simulink model "lineprotsys"  (Simulink 9.3)
settings: Solver=ode23tb  StartTime=0.0  StopTime=0.15  RelTol=1e-3  AbsTol=20e-6
values from neighbouring files (symbols this model uses):
  n = abs(fix(dif/360))    [DE_12.m]
undefined symbols (not defined in the file or in its folder): b, flagc, m, minx
libraries: elements x42, Relay_Elements x9
settings Model: Creator=Dr. Lotfifard  LastModifiedBy=renji  ExtModeTrigMode=oneshot  ExtModeArmWhenConnect=off
settings SolverCC: AutoScaleAbsTol=off  MaxOrder=2
settings DataIOCC: LimitDataPoints=on
settings OptimizationCC: BlockReduction=off  BooleanDataType=off  ExpressionDepthLimit=2147483647
settings DebuggingCC: SaveWithParameterizedLinksMsg=none  SignalResolutionControl=TryResolveAllWithWarning  MultiTaskDSMMsg=warning  MultiTaskCondExecSysMsg=none  StateNameClashWarn=warning
settings HardwareCC: TargetUnknown=on
settings RTWCC: TemplateMakefile=grt_unix.tmf
settings GRTTargetCC: GeneratePreprocessorConditionals=Disable all
settings SimscapeCC: SimscapeNormalizeSystem=off
settings ConfigurationSet: Description=SimMechanics 2G

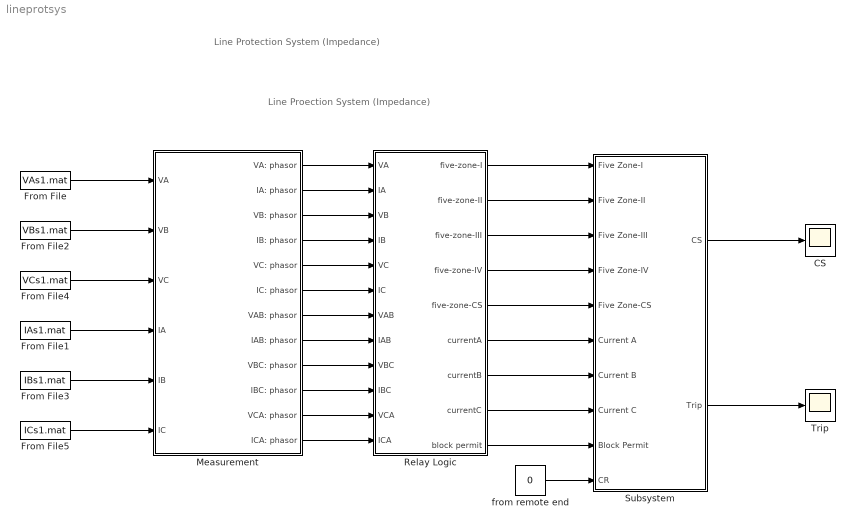
== system lineprotsys ==
  note: Line Protection System (Impedance)
  note: Line Proection System (Impedance)
  CS : Scope
  From File : FromFile  FileName=VAs1.mat  SampleTime=0
  From File1 : FromFile  FileName=IAs1.mat  SampleTime=0
  From File2 : FromFile  FileName=VBs1.mat  SampleTime=0
  From File3 : FromFile  FileName=IBs1.mat  SampleTime=0
  From File4 : FromFile  FileName=VCs1.mat  SampleTime=0
  From File5 : FromFile  FileName=ICs1.mat  SampleTime=0
  Measurement : Subsystem
  Relay Logic : Subsystem  mask{RelayZones=[70 90 100 120 60], fDetectZone=10, PolarZangle=pi/4, PolarZset=2, PowerSwingDetect=[0.05 1 2 5 10], ICtime=0.1, ICpu=0.005, CDang1=170, CDang2=0}
      mask prompts: RelayZones "Relay Zones [z1 z2 z3 z4 zb]"; fDetectZone "Fault Detection Zone (lenght and width)"; PolarZangle "Memory Polariztion: Zangle"; PolarZset "Memory Polariztion: Zsetting"; PowerSwingDetect "Power Swing Detection: [DeltT zs11 zs12 zs21 zs22"; ICtime "Inverse Current: time parameter"; ICpu "Inverse Current: pick up value"; CDang1 "Current Direction: angle1"; CDang2 "Current Direction: angle2"
  Subsystem : Subsystem
  Trip : Scope
  from remote end : Constant  Value=0
  wires:
  From File5/1 -> Measurement/6(IC)
  From File3/1 -> Measurement/5(IB)
  From File1/1 -> Measurement/4(IA)
  From File4/1 -> Measurement/3(VC)
  From File2/1 -> Measurement/2(VB)
  From File/1 -> Measurement/1(VA)
  Measurement/1(VA: phasor) -> Relay Logic/1(VA)
  Measurement/2(IA: phasor) -> Relay Logic/2(IA)
  Measurement/3(VB: phasor) -> Relay Logic/3(VB)
  Measurement/4(IB: phasor) -> Relay Logic/4(IB)
  Measurement/5(VC: phasor) -> Relay Logic/5(VC)
  Measurement/6(IC: phasor) -> Relay Logic/6(IC)
  Measurement/7(VAB: phasor) -> Relay Logic/7(VAB)
  Measurement/8(IAB: phasor) -> Relay Logic/8(IAB)
  Measurement/9(VBC: phasor) -> Relay Logic/9(VBC)
  Measurement/10(IBC: phasor) -> Relay Logic/10(IBC)
  Measurement/11(VCA: phasor) -> Relay Logic/11(VCA)
  Measurement/12(ICA: phasor) -> Relay Logic/12(ICA)
  Relay Logic/1(five-zone-I) -> Subsystem/1(Five Zone-I)
  Relay Logic/2(five-zone-II) -> Subsystem/2(Five Zone-II)
  Relay Logic/3(five-zone-III) -> Subsystem/3(Five Zone-III)
  Relay Logic/4(five-zone-IV) -> Subsystem/4(Five Zone-IV)
  Relay Logic/5(five-zone-CS) -> Subsystem/5(Five Zone-CS)
  Relay Logic/6(currentA) -> Subsystem/6(Current A)
  Relay Logic/7(currentB) -> Subsystem/7(Current B)
  Relay Logic/8(currentC) -> Subsystem/8(Current C)
  Relay Logic/9(block permit) -> Subsystem/9(Block Permit)
  from remote end/1 -> Subsystem/10(CR)
  Subsystem/1(CS) -> CS/1
  Subsystem/2(Trip) -> Trip/1

== system lineprotsys/Measurement ==
  note: Measurement Block
  VA : Inport
  VB : Inport  Port=2
  VC : Inport  Port=3
  IA : Inport  Port=4
  IB : Inport  Port=5
  IC : Inport  Port=6
  Input Signal Board : Subsystem
  Phase-phase Measurements : Subsystem
  Single Phase Measurements : Subsystem
  VA: phasor : Outport
  IA: phasor : Outport  Port=2
  VB: phasor : Outport  Port=3
  IB: phasor : Outport  Port=4
  VC: phasor : Outport  Port=5
  IC: phasor : Outport  Port=6
  VAB: phasor : Outport  Port=7
  IAB: phasor : Outport  Port=8
  VBC: phasor : Outport  Port=9
  IBC: phasor : Outport  Port=10
  VCA: phasor : Outport  Port=11
  ICA: phasor : Outport  Port=12
  wires:
  Phase-phase Measurements/1(VAB: phasor) -> VAB: phasor/1
  Phase-phase Measurements/6(ICA: phasor) -> ICA: phasor/1
  Phase-phase Measurements/4(IBC: phasor) -> IBC: phasor/1
  Phase-phase Measurements/2(IAB: phasor) -> IAB: phasor/1
  Phase-phase Measurements/3(VBC: phasor) -> VBC: phasor/1
  Phase-phase Measurements/5(VCA: phasor) -> VCA: phasor/1
  Single Phase Measurements/5(VC: phasor) -> VC: phasor/1
  Single Phase Measurements/6(IC: phasor) -> IC: phasor/1
  IC/1 -> Input Signal Board/6(IC)
  IB/1 -> Input Signal Board/5(IB)
  VC/1 -> Input Signal Board/3(VC)
  IA/1 -> Input Signal Board/4(IA)
  Single Phase Measurements/2(IA: phasor) -> IA: phasor/1
  Single Phase Measurements/3(VB: phasor) -> VB: phasor/1
  Single Phase Measurements/4(IB: phasor) -> IB: phasor/1
  VA/1 -> Input Signal Board/1(VA)
  Single Phase Measurements/1(VA: phasor) -> VA: phasor/1
  VB/1 -> Input Signal Board/2(VB)

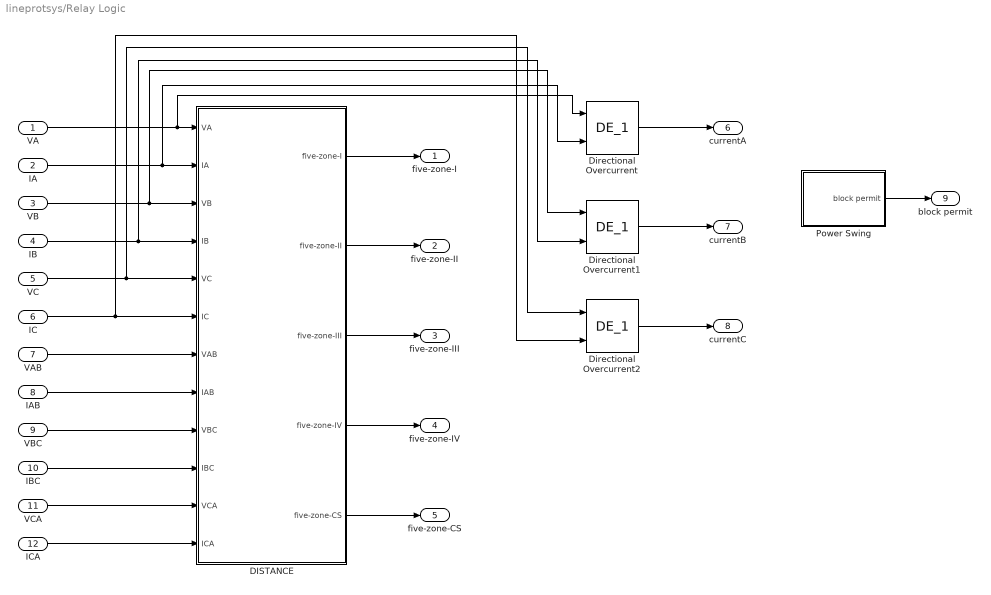
== system lineprotsys/Relay Logic ==
  VA : Inport
  IA : Inport  Port=2
  VB : Inport  Port=3
  IB : Inport  Port=4
  VC : Inport  Port=5
  IC : Inport  Port=6
  VAB : Inport  Port=7
  IAB : Inport  Port=8
  VBC : Inport  Port=9
  IBC : Inport  Port=10
  VCA : Inport  Port=11
  ICA : Inport  Port=12
  "  Directional Overcurrent" : Relay_Elements/  DE_1  alpha=CDang1  beta=CDang2  fs=20*60
  "  Directional Overcurrent1" : Relay_Elements/  DE_1  alpha=CDang1  beta=CDang2  fs=20*60
  "  Directional Overcurrent2" : Relay_Elements/  DE_1  alpha=CDang1  beta=CDang2  fs=20*60
  DISTANCE : Subsystem
  Power Swing : Subsystem  mask{Tswing=PowerSwingDetect(1)}
      mask prompts: Tswing "T Power Swing (sec)"
  five-zone-I : Outport
  five-zone-II : Outport  Port=2
  five-zone-III : Outport  Port=3
  five-zone-IV : Outport  Port=4
  five-zone-CS : Outport  Port=5
  currentA : Outport  Port=6
  currentB : Outport  Port=7
  currentC : Outport  Port=8
  block permit : Outport  Port=9
  wires:
  DISTANCE/1(five-zone-I) -> five-zone-I/1
  DISTANCE/2(five-zone-II) -> five-zone-II/1
  DISTANCE/3(five-zone-III) -> five-zone-III/1
  DISTANCE/4(five-zone-IV) -> five-zone-IV/1
  DISTANCE/5(five-zone-CS) -> five-zone-CS/1
  "  Directional Overcurrent1"/1 -> currentB/1
  "  Directional Overcurrent"/1 -> currentA/1
  "  Directional Overcurrent2"/1 -> currentC/1
  Power Swing/1(block permit) -> block permit/1
  VA/1 -> "  Directional Overcurrent"/1, DISTANCE/1(VA)
  VB/1 -> "  Directional Overcurrent1"/1, DISTANCE/3(VB)
  IB/1 -> "  Directional Overcurrent1"/2, DISTANCE/4(IB)
  VC/1 -> "  Directional Overcurrent2"/1, DISTANCE/5(VC)
  IC/1 -> "  Directional Overcurrent2"/2, DISTANCE/6(IC)
  VAB/1 -> DISTANCE/7(VAB)
  IAB/1 -> DISTANCE/8(IAB)
  VBC/1 -> DISTANCE/9(VBC)
  IBC/1 -> DISTANCE/10(IBC)
  VCA/1 -> DISTANCE/11(VCA)
  ICA/1 -> DISTANCE/12(ICA)
  IA/1 -> "  Directional Overcurrent"/2, DISTANCE/2(IA)

== system lineprotsys/Subsystem ==
  Five Zone-I : Inport
  Five Zone-II : Inport  Port=2
  Five Zone-III : Inport  Port=3
  Five Zone-IV : Inport  Port=4
  Five Zone-CS : Inport  Port=5
  Current A : Inport  Port=6
  Current B : Inport  Port=7
  Current C : Inport  Port=8
  Block Permit : Inport  Port=9
  CR : Inport  Port=10
  1 : Logic  Operator=OR  Inputs=4  AllPortsSameDT=off
  2 : Logic  Inputs=4
  3 : Logic  Operator=OR  Inputs=3  AllPortsSameDT=off
  4 : Logic  Operator=OR
  Not : Logic  Operator=NOT  AllPortsSameDT=off  OutDataTypeStr=boolean
  Not1 : Logic  Operator=NOT  AllPortsSameDT=off  OutDataTypeStr=boolean
  Not2 : Logic  Operator=NOT  AllPortsSameDT=off  OutDataTypeStr=boolean
  CS : Outport
  Trip : Outport  Port=2
  wires:
  Five Zone-II/1 -> 1/2
  Five Zone-IV/1 -> 1/4
  Five Zone-I/1 -> 1/1
  Current A/1 -> 3/1
  Current C/1 -> 3/3
  3/1 -> 4/2
  Five Zone-III/1 -> 1/3
  Current B/1 -> 3/2
  1/1 -> 4/1
  Block Permit/1 -> Not/1
  CR/1 -> Not2/1
  Not2/1 -> 2/4
  Not/1 -> 2/3
  Five Zone-CS/1 -> Not1/1
  Not1/1 -> CS/1, 2/2
  2/1 -> Trip/1
  4/1 -> 2/1

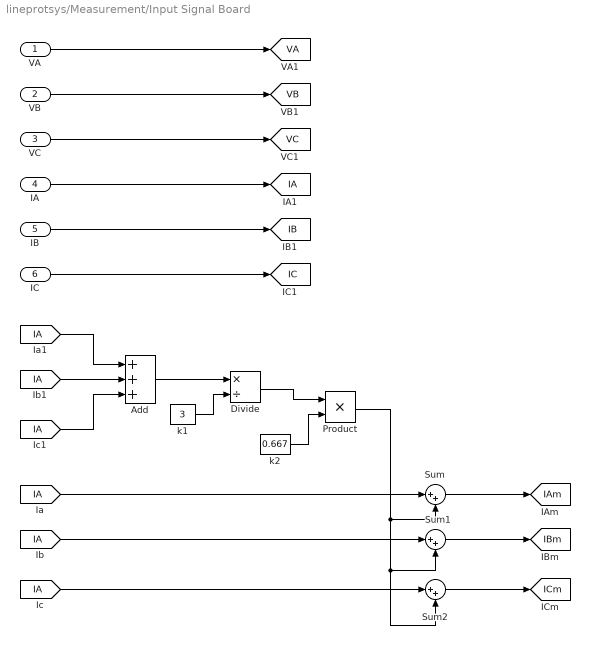
== system lineprotsys/Measurement/Input Signal Board ==
  VA : Inport
  VB : Inport  Port=2
  VC : Inport  Port=3
  IA : Inport  Port=4
  IB : Inport  Port=5
  IC : Inport  Port=6
  Add : Sum  Inputs=+++
  Divide : Product  Inputs=*/
  Product : Product
  Sum : Sum  Inputs=|++
  Sum1 : Sum  Inputs=|++
  Sum2 : Sum  Inputs=|++
  k1 : Constant  Value=3
  k2 : Constant  Value=0.667
  tag scope: IA=global, IAm=global, IB=global, IBm=global, IC=global, ICm=global, VA=global, VB=global, VC=global
  wires:
  Add/1 -> Divide/1
  k1/1 -> Divide/2
  Divide/1 -> Product/1
  VC/1 -> [VC]
  k2/1 -> Product/2
  VB/1 -> [VB]
  IA/1 -> [IA]
  IB/1 -> [IB]
  IC/1 -> [IC]
  [IA] -> Add/2
  [IA] -> Add/1
  [IA] -> Add/3
  VA/1 -> [VA]
  Sum2/1 -> [ICm]
  Sum1/1 -> [IBm]
  Sum/1 -> [IAm]
  [IA] -> Sum2/1
  [IA] -> Sum1/1
  [IA] -> Sum/1
  Product/1 -> Sum/2, Sum1/2, Sum2/2

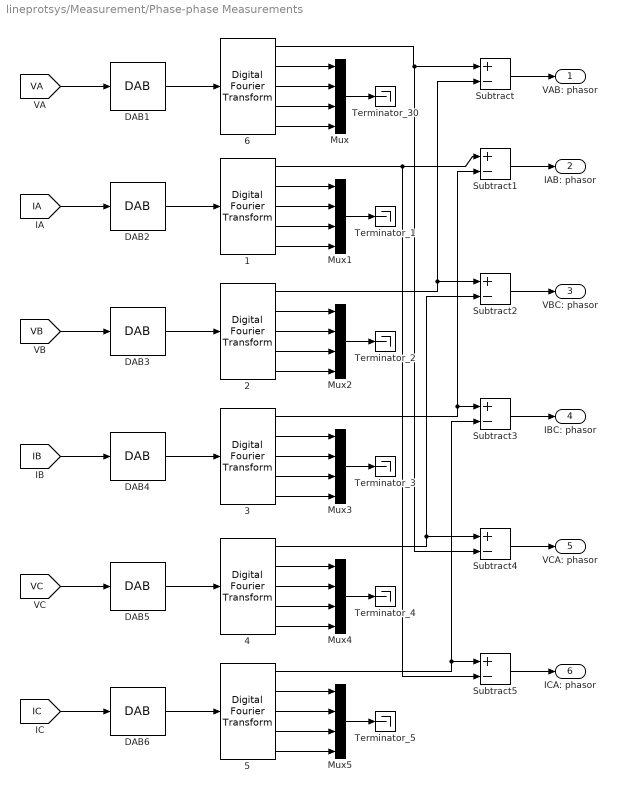
== system lineprotsys/Measurement/Phase-phase Measurements ==
   {1..6} (6 alike) : elements/   fo=60  window_size=32  harmonic=[1 2 3 4 5]
  DAB{1..6} (6 alike) : elements/DAB  filter=off  approx=Bessel  order=2  numerator=[]  denominator=[]  freq=360  resdis=off  vertres=12  xmax=10  winsize=32  G=1.0  fs=60*32
  Mux{,1..5} (6 alike) : Mux
  Subtract{,1..5} (6 alike) : Sum  Inputs=+-
  Terminator_{1..5,30} (6 alike) : Terminator
  VAB: phasor : Outport
  IAB: phasor : Outport  Port=2
  VBC: phasor : Outport  Port=3
  IBC: phasor : Outport  Port=4
  VCA: phasor : Outport  Port=5
  ICA: phasor : Outport  Port=6
  wires:
  " 4"/5 -> Mux4/4
  Mux4/1 -> Terminator_4/1
  DAB5/1 -> " 4"/1
  " 2"/3 -> Mux2/2
  " 2"/2 -> Mux2/1
  " 2"/5 -> Mux2/4
  DAB3/1 -> " 2"/1
  " 2"/4 -> Mux2/3
  Mux2/1 -> Terminator_2/1
  " 4"/2 -> Mux4/1
  " 4"/3 -> Mux4/2
  " 4"/4 -> Mux4/3
  " 1"/2 -> Mux1/1
  " 1"/3 -> Mux1/2
  " 1"/4 -> Mux1/3
  " 1"/5 -> Mux1/4
  Mux1/1 -> Terminator_1/1
  DAB2/1 -> " 1"/1
  DAB1/1 -> " 6"/1
  " 5"/3 -> Mux5/2
  " 5"/2 -> Mux5/1
  " 5"/4 -> Mux5/3
  " 5"/5 -> Mux5/4
  Mux5/1 -> Terminator_5/1
  DAB6/1 -> " 5"/1
  " 6"/5 -> Mux/4
  " 6"/3 -> Mux/2
  Mux/1 -> Terminator_30/1
  Mux3/1 -> Terminator_3/1
  " 3"/3 -> Mux3/2
  DAB4/1 -> " 3"/1
  " 3"/2 -> Mux3/1
  " 3"/4 -> Mux3/3
  " 3"/5 -> Mux3/4
  " 6"/4 -> Mux/3
  " 6"/2 -> Mux/1
  [VA] -> DAB1/1
  [IA] -> DAB2/1
  [VB] -> DAB3/1
  [IB] -> DAB4/1
  [VC] -> DAB5/1
  [IC] -> DAB6/1
  " 6"/1 -> Subtract4/2, Subtract/1
  " 2"/1 -> Subtract2/1, Subtract/2
  Subtract/1 -> VAB: phasor/1
  " 1"/1 -> Subtract5/2, Subtract1/1
  " 3"/1 -> Subtract3/1, Subtract1/2
  " 4"/1 -> Subtract4/1, Subtract2/2
  Subtract2/1 -> VBC: phasor/1
  Subtract1/1 -> IAB: phasor/1
  Subtract3/1 -> IBC: phasor/1
  Subtract4/1 -> VCA: phasor/1
  Subtract5/1 -> ICA: phasor/1
  " 5"/1 -> Subtract5/1, Subtract3/2

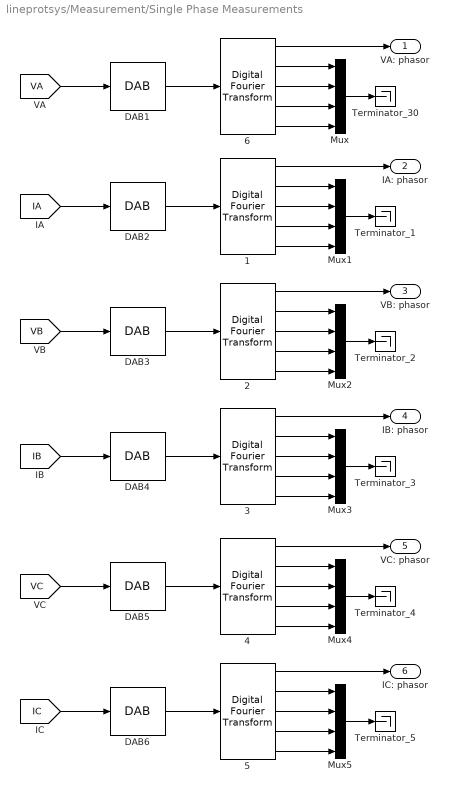
== system lineprotsys/Measurement/Single Phase Measurements ==
   {1..6} (6 alike) : elements/   fo=60  window_size=32  harmonic=[1 2 3 4 5]
  DAB{1..6} (6 alike) : elements/DAB  filter=off  approx=Bessel  order=2  numerator=[]  denominator=[]  freq=360  resdis=off  vertres=12  xmax=10  winsize=32  G=1.0  fs=60*32
  Mux{,1..5} (6 alike) : Mux
  Terminator_{1..5,30} (6 alike) : Terminator
  VA: phasor : Outport
  IA: phasor : Outport  Port=2
  VB: phasor : Outport  Port=3
  IB: phasor : Outport  Port=4
  VC: phasor : Outport  Port=5
  IC: phasor : Outport  Port=6
  wires:
  " 4"/1 -> VC: phasor/1
  " 4"/5 -> Mux4/4
  Mux4/1 -> Terminator_4/1
  DAB5/1 -> " 4"/1
  " 2"/3 -> Mux2/2
  " 2"/2 -> Mux2/1
  " 2"/5 -> Mux2/4
  DAB3/1 -> " 2"/1
  " 2"/4 -> Mux2/3
  " 2"/1 -> VB: phasor/1
  Mux2/1 -> Terminator_2/1
  " 4"/2 -> Mux4/1
  " 4"/3 -> Mux4/2
  " 4"/4 -> Mux4/3
  " 1"/2 -> Mux1/1
  " 1"/3 -> Mux1/2
  " 1"/4 -> Mux1/3
  " 1"/5 -> Mux1/4
  Mux1/1 -> Terminator_1/1
  " 1"/1 -> IA: phasor/1
  DAB2/1 -> " 1"/1
  DAB1/1 -> " 6"/1
  " 5"/1 -> IC: phasor/1
  " 5"/3 -> Mux5/2
  " 5"/2 -> Mux5/1
  " 5"/4 -> Mux5/3
  " 5"/5 -> Mux5/4
  Mux5/1 -> Terminator_5/1
  DAB6/1 -> " 5"/1
  " 6"/5 -> Mux/4
  " 6"/3 -> Mux/2
  Mux/1 -> Terminator_30/1
  Mux3/1 -> Terminator_3/1
  " 3"/3 -> Mux3/2
  " 3"/1 -> IB: phasor/1
  DAB4/1 -> " 3"/1
  " 6"/1 -> VA: phasor/1
  " 3"/2 -> Mux3/1
  " 3"/4 -> Mux3/3
  " 3"/5 -> Mux3/4
  " 6"/4 -> Mux/3
  " 6"/2 -> Mux/1
  [VA] -> DAB1/1
  [IA] -> DAB2/1
  [VB] -> DAB3/1
  [IB] -> DAB4/1
  [VC] -> DAB5/1
  [IC] -> DAB6/1

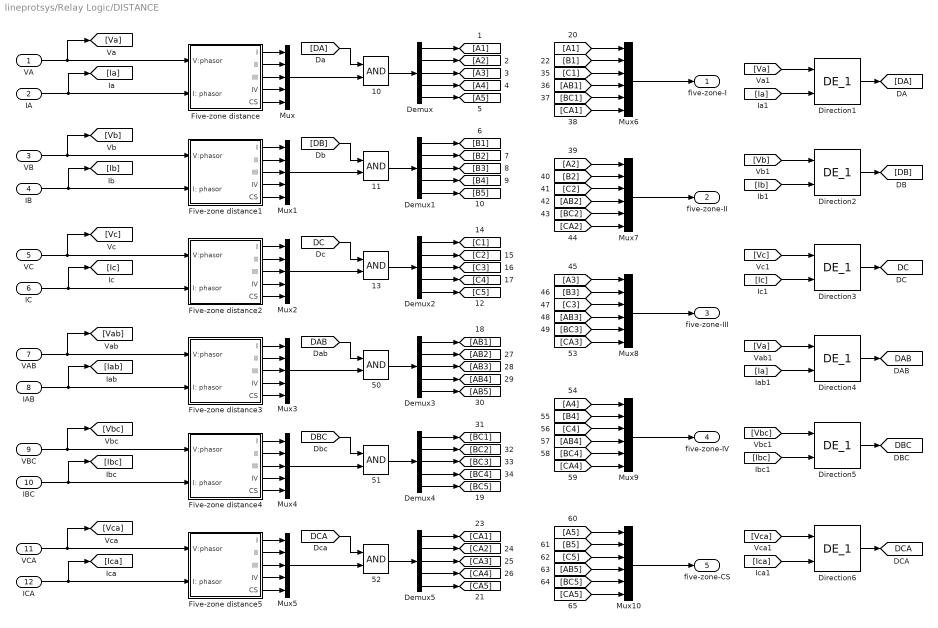
== system lineprotsys/Relay Logic/DISTANCE ==
  VA : Inport
  IA : Inport  Port=2
  VB : Inport  Port=3
  IB : Inport  Port=4
  VC : Inport  Port=5
  IC : Inport  Port=6
  VAB : Inport  Port=7
  IAB : Inport  Port=8
  VBC : Inport  Port=9
  IBC : Inport  Port=10
  VCA : Inport  Port=11
  ICA : Inport  Port=12
    Direction{1..6} (6 alike) : Relay_Elements/  DE_1  alpha=CDang1  beta=CDang2  fs=20*60
  "10 " : Logic
  {11,13,50..52} (5 alike) : Logic
  Demux{,1..5} (6 alike) : Demux  Outputs=5
  Five-zone distance : Subsystem
  Five-zone distance1 : Subsystem
  Five-zone distance2 : Subsystem
  Five-zone distance3 : Subsystem
  Five-zone distance4 : Subsystem
  Five-zone distance5 : Subsystem
  Mux{,1..5} (6 alike) : Mux  Inputs=5
  Mux{6..10} (5 alike) : Mux  Inputs=6
  five-zone-I : Outport
  five-zone-II : Outport  Port=2
  five-zone-III : Outport  Port=3
  five-zone-IV : Outport  Port=4
  five-zone-CS : Outport  Port=5
  tag scope: DAB=global, DBC=global, DC=global, DCA=global
  wires:
  VB/1 -> Five-zone distance1/1(V:phasor), [Vb]
  IB/1 -> Five-zone distance1/2(I: phasor), [Ib]
  [DB] -> 11/1
  Demux1/1 -> [B1]
  Demux1/3 -> [B3]
  Five-zone distance1/4(IV) -> Mux1/4
  Five-zone distance1/5(CS) -> Mux1/5
  Mux1/1 -> 11/2
  Demux1/2 -> [B2]
  Demux1/5 -> [B5]
  Five-zone distance1/1(I) -> Mux1/1
  Five-zone distance1/3(III) -> Mux1/3
  11/1 -> Demux1/1
  Five-zone distance1/2(II) -> Mux1/2
  Demux1/4 -> [B4]
  Five-zone distance/2(II) -> Mux/2
  Five-zone distance/5(CS) -> Mux/5
  Five-zone distance/4(IV) -> Mux/4
  "  Direction1"/1 -> [DA]
  Five-zone distance/1(I) -> Mux/1
  IA/1 -> [Ia], Five-zone distance/2(I: phasor)
  VA/1 -> [Va], Five-zone distance/1(V:phasor)
  Demux/3 -> [A3]
  Demux/5 -> [A5]
  Demux/4 -> [A4]
  [B2] -> Mux7/2
  [AB2] -> Mux7/4
  [C2] -> Mux7/3
  [CA2] -> Mux7/6
  [A2] -> Mux7/1
  Mux7/1 -> five-zone-II/1
  [BC2] -> Mux7/5
  [B1] -> Mux6/2
  [CA1] -> Mux6/6
  "10 "/1 -> Demux/1
  [BC1] -> Mux6/5
  [A1] -> Mux6/1
  Demux/1 -> [A1]
  Demux/2 -> [A2]
  [C1] -> Mux6/3
  [AB1] -> Mux6/4
  [A3] -> Mux8/1
  [B3] -> Mux8/2
  [C3] -> Mux8/3
  [CA3] -> Mux8/6
  [AB3] -> Mux8/4
  [BC3] -> Mux8/5
  Mux8/1 -> five-zone-III/1
  Mux10/1 -> five-zone-CS/1
  [A5] -> Mux10/1
  [C5] -> Mux10/3
  [CA5] -> Mux10/6
  [B5] -> Mux10/2
  [BC5] -> Mux10/5
  [AB5] -> Mux10/4
  [B4] -> Mux9/2
  [CA4] -> Mux9/6
  [BC4] -> Mux9/5
  [AB4] -> Mux9/4
  [A4] -> Mux9/1
  [C4] -> Mux9/3
  Mux9/1 -> five-zone-IV/1
  Mux2/1 -> 13/2
  Demux2/3 -> [C3]
  Five-zone distance2/1(I) -> Mux2/1
  Demux2/1 -> [C1]
  VC/1 -> Five-zone distance2/1(V:phasor), [Vc]
  Five-zone distance2/3(III) -> Mux2/3
  IC/1 -> Five-zone distance2/2(I: phasor), [Ic]
  [DC] -> 13/1
  Five-zone distance2/5(CS) -> Mux2/5
  Five-zone distance2/2(II) -> Mux2/2
  13/1 -> Demux2/1
  Five-zone distance2/4(IV) -> Mux2/4
  Demux2/2 -> [C2]
  Demux2/5 -> [C5]
  Demux2/4 -> [C4]
  Five-zone distance/3(III) -> Mux/3
  [DA] -> "10 "/1
  Mux/1 -> "10 "/2
  Five-zone distance5/4(IV) -> Mux5/4
  Mux5/1 -> 52/2
  IAB/1 -> Five-zone distance3/2(I: phasor), [Iab]
  Five-zone distance3/1(I) -> Mux3/1
  Demux4/5 -> [BC5]
  Demux4/4 -> [BC4]
  Demux3/5 -> [AB5]
  Five-zone distance3/3(III) -> Mux3/3
  Demux3/4 -> [AB4]
  Five-zone distance5/5(CS) -> Mux5/5
  [DCA] -> 52/1
  Demux5/5 -> [CA5]
  Demux3/1 -> [AB1]
  Five-zone distance3/4(IV) -> Mux3/4
  Five-zone distance3/5(CS) -> Mux3/5
  [DAB] -> 50/1
  Demux3/3 -> [AB3]
  IBC/1 -> Five-zone distance4/2(I: phasor), [Ibc]
  Mux4/1 -> 51/2
  50/1 -> Demux3/1
  Demux4/1 -> [BC1]
  Five-zone distance5/1(I) -> Mux5/1
  52/1 -> Demux5/1
  Demux5/1 -> [CA1]
  51/1 -> Demux4/1
  VAB/1 -> Five-zone distance3/1(V:phasor), [Vab]
  Demux4/3 -> [BC3]
  Demux4/2 -> [BC2]
  Five-zone distance3/2(II) -> Mux3/2
  VBC/1 -> Five-zone distance4/1(V:phasor), [Vbc]
  Mux3/1 -> 50/2
  Demux3/2 -> [AB2]
  Five-zone distance5/2(II) -> Mux5/2
  ICA/1 -> Five-zone distance5/2(I: phasor), [Ica]
  Demux5/2 -> [CA2]
  Five-zone distance5/3(III) -> Mux5/3
  Demux5/3 -> [CA3]
  [DBC] -> 51/1
  Demux5/4 -> [CA4]
  VCA/1 -> Five-zone distance5/1(V:phasor), [Vca]
  [Va] -> "  Direction4"/1
  "  Direction4"/1 -> [DAB]
  [Ia] -> "  Direction4"/2
  [Ica] -> "  Direction6"/2
  [Vca] -> "  Direction6"/1
  "  Direction6"/1 -> [DCA]
  [Va] -> "  Direction1"/1
  [Ia] -> "  Direction1"/2
  [Vc] -> "  Direction3"/1
  [Ic] -> "  Direction3"/2
  "  Direction3"/1 -> [DC]
  [Vbc] -> "  Direction5"/1
  "  Direction5"/1 -> [DBC]
  [Ibc] -> "  Direction5"/2
  Mux6/1 -> five-zone-I/1
  "  Direction2"/1 -> [DB]
  [Ib] -> "  Direction2"/2
  [Vb] -> "  Direction2"/1
  Five-zone distance4/1(I) -> Mux4/1
  Five-zone distance4/2(II) -> Mux4/2
  Five-zone distance4/3(III) -> Mux4/3
  Five-zone distance4/4(IV) -> Mux4/4
  Five-zone distance4/5(CS) -> Mux4/5

== system lineprotsys/Relay Logic/Power Swing ==
  " 3" : Terminator
  " 4" : Terminator
  " 6" : Terminator
  4 : Logic  Operator=OR
  Subsystem : Subsystem
  Z: power swing : Subsystem  mask(Zone Comparator){typez=Free expression, z1=[0.2 0.2;-0.2 0.2; -0.2 -0.2;0.2 -0.2], z2=[0 0;1 1; -1 1;0 0], z3=[1 1;-1 1;-1 -1;1 -1], z4=[0 0;0 0;0 0;0 0], zr=[0 0;0 0;0 0;0 0], fs=32*60}
      mask prompts: typez "shape"; z1 "Zone 1"; z2 "Zone 2"; z3 "Zone 3"; z4 "Zone 4"; zr "Reverse Zone"; fs "Sampling frecuency (Hz):"
      mask help: This block performs the zone comparison. Its inputs are the resistance and reactance signals. Four forward and one backward zones are implemented. The output that corresponds to the zone where the impedance is located is set to one while the rest of the outputs are zero Either the mho or free expression characteristics may be set. For the mho characteristic, the zones are defined by specifying the center of each circle (all the circles are tangent to the origin). For the free expression, arrays with consecutive vertices specify the polygons for each zone.
      mask init:
      | zc1;
      mask Help: web(['file:///' which('zc.html')]);
      mask TypeOptions typez: Mho characteristic | Free expression
      mask Display:
      | plot(x1(:,1),x1(:,2));
      | plot(x2(:,1),x2(:,2));
      | plot(x3(:,1),x3(:,2));
      | plot(x4(:,1),x4(:,2));
      | plot(xr(:,1),xr(:,2));
  block permit : Outport
  wires:
  Z: power swing/3(3) -> " 3"/1
  Z: power swing/2(2) -> 4/2
  Z: power swing/1(1) -> Subsystem/1(Z1), 4/1
  [ZA] -> Z: power swing/1(Z)
  Z: power swing/5(R) -> " 6"/1
  Z: power swing/4(4) -> " 4"/1
  4/1 -> Subsystem/2(Z2)
  Subsystem/1(block) -> block permit/1

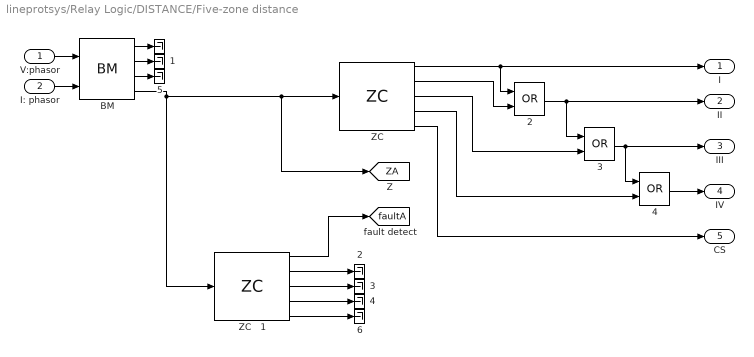
== system lineprotsys/Relay Logic/DISTANCE/Five-zone distance ==
  V:phasor : Inport
  I: phasor : Inport  Port=2
   {,1..6} (7 alike) : Terminator
  "2 " : Logic  Operator=OR
  3 : Logic  Operator=OR
  4 : Logic  Operator=OR
  BM : elements/BM  tpostv=none  plenv=4  tposti=none  pleni=4  tposts=none  plens=4  tpostz=none  plenz=4
  "ZC   " : elements/ZC     typez=Free expression  z1="[0  0; RelayZones(1) 0; RelayZones(1) RelayZones(1); 0 RelayZones(1)]"  z2="[0  0; RelayZones(2) 0; RelayZones(2) RelayZones(2); 0 RelayZones(2)]"  z3="[0  0; RelayZones(3) 0; RelayZones(3) RelayZones(3); 0 RelayZones(3)]"  z4="[0  0; RelayZones(4) 0; RelayZones(4) RelayZones(4); 0 RelayZones(4)]"  zr="[0  0; -RelayZones(5) 0; -RelayZones(5) -RelayZones(5); 0 -RelayZones(5)]"  fs=32*60
  ZC   1 : elements/ZC     typez=Free expression  z1="[0  0; RelayZones(1) 0; RelayZones(1) RelayZones(1); 0 RelayZones(1)]"  z2="[0  0; RelayZones(2) 0; RelayZones(2) RelayZones(2); 0 RelayZones(2)]"  z3="[0  0; RelayZones(3) 0; RelayZones(3) RelayZones(3); 0 RelayZones(3)]"  z4="[0  0; RelayZones(4) 0; RelayZones(4) RelayZones(4); 0 RelayZones(4)]"  zr="[0  0; -RelayZones(5) 0; -RelayZones(5) -RelayZones(5); 0 -RelayZones(5)]"  fs=32*60
  I : Outport
  II : Outport  Port=2
  III : Outport  Port=3
  IV : Outport  Port=4
  CS : Outport  Port=5
  tag scope: ZA=global, faultA=global
  wires:
  BM/1 -> " "/1
  BM/2 -> " 1"/1
  BM/3 -> " 5"/1
  V:phasor/1 -> BM/1
  I: phasor/1 -> BM/2
  BM/4 -> ZC   1/1, [ZA], "ZC   "/1
  ZC   1/2 -> " 2"/1
  ZC   1/3 -> " 3"/1
  ZC   1/4 -> " 4"/1
  ZC   1/5 -> " 6"/1
  "2 "/1 -> II/1, 3/1
  3/1 -> 4/1, III/1
  4/1 -> IV/1
  "ZC   "/5 -> CS/1
  "ZC   "/4 -> 4/2
  "ZC   "/3 -> 3/2
  "ZC   "/2 -> "2 "/2
  "ZC   "/1 -> "2 "/1, I/1
  ZC   1/1 -> [faultA]

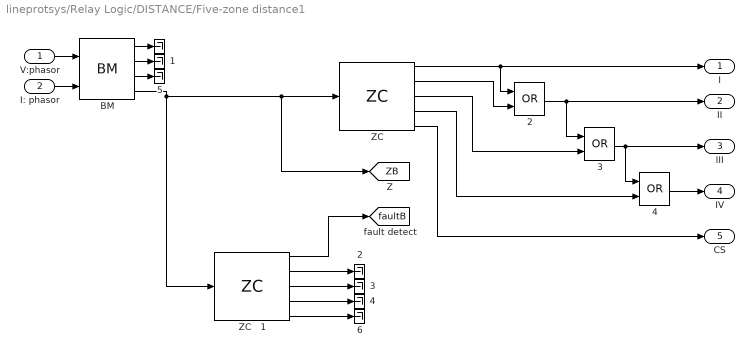
== system lineprotsys/Relay Logic/DISTANCE/Five-zone distance1 ==
  V:phasor : Inport
  I: phasor : Inport  Port=2
   {,1..6} (7 alike) : Terminator
  "2 " : Logic  Operator=OR
  3 : Logic  Operator=OR
  4 : Logic  Operator=OR
  BM : elements/BM  tpostv=none  plenv=4  tposti=none  pleni=4  tposts=none  plens=4  tpostz=none  plenz=4
  "ZC   " : elements/ZC     typez=Free expression  z1="[0  0; RelayZones(1) 0; RelayZones(1) RelayZones(1); 0 RelayZones(1)]"  z2="[0  0; RelayZones(2) 0; RelayZones(2) RelayZones(2); 0 RelayZones(2)]"  z3="[0  0; RelayZones(3) 0; RelayZones(3) RelayZones(3); 0 RelayZones(3)]"  z4="[0  0; RelayZones(4) 0; RelayZones(4) RelayZones(4); 0 RelayZones(4)]"  zr="[0  0; -RelayZones(5) 0; -RelayZones(5) -RelayZones(5); 0 -RelayZones(5)]"  fs=32*60
  ZC   1 : elements/ZC     typez=Free expression  z1="[0  0; RelayZones(1) 0; RelayZones(1) RelayZones(1); 0 RelayZones(1)]"  z2="[0  0; RelayZones(2) 0; RelayZones(2) RelayZones(2); 0 RelayZones(2)]"  z3="[0  0; RelayZones(3) 0; RelayZones(3) RelayZones(3); 0 RelayZones(3)]"  z4="[0  0; RelayZones(4) 0; RelayZones(4) RelayZones(4); 0 RelayZones(4)]"  zr="[0  0; -RelayZones(5) 0; -RelayZones(5) -RelayZones(5); 0 -RelayZones(5)]"  fs=32*60
  I : Outport
  II : Outport  Port=2
  III : Outport  Port=3
  IV : Outport  Port=4
  CS : Outport  Port=5
  tag scope: ZB=global, faultB=global
  wires:
  BM/1 -> " "/1
  BM/2 -> " 1"/1
  BM/3 -> " 5"/1
  V:phasor/1 -> BM/1
  I: phasor/1 -> BM/2
  BM/4 -> ZC   1/1, [ZB], "ZC   "/1
  ZC   1/2 -> " 2"/1
  ZC   1/3 -> " 3"/1
  ZC   1/4 -> " 4"/1
  ZC   1/5 -> " 6"/1
  "2 "/1 -> II/1, 3/1
  3/1 -> 4/1, III/1
  4/1 -> IV/1
  "ZC   "/5 -> CS/1
  "ZC   "/4 -> 4/2
  "ZC   "/3 -> 3/2
  "ZC   "/2 -> "2 "/2
  "ZC   "/1 -> "2 "/1, I/1
  ZC   1/1 -> [faultB]

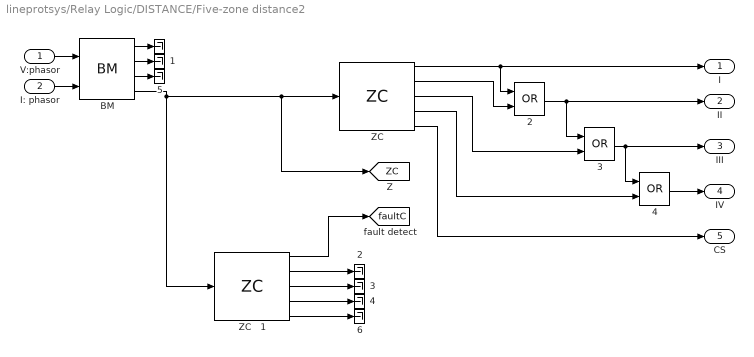
== system lineprotsys/Relay Logic/DISTANCE/Five-zone distance2 ==
  V:phasor : Inport
  I: phasor : Inport  Port=2
   {,1..6} (7 alike) : Terminator
  "2 " : Logic  Operator=OR
  3 : Logic  Operator=OR
  4 : Logic  Operator=OR
  BM : elements/BM  tpostv=none  plenv=4  tposti=none  pleni=4  tposts=none  plens=4  tpostz=none  plenz=4
  "ZC   " : elements/ZC     typez=Free expression  z1="[0  0; RelayZones(1) 0; RelayZones(1) RelayZones(1); 0 RelayZones(1)]"  z2="[0  0; RelayZones(2) 0; RelayZones(2) RelayZones(2); 0 RelayZones(2)]"  z3="[0  0; RelayZones(3) 0; RelayZones(3) RelayZones(3); 0 RelayZones(3)]"  z4="[0  0; RelayZones(4) 0; RelayZones(4) RelayZones(4); 0 RelayZones(4)]"  zr="[0  0; -RelayZones(5) 0; -RelayZones(5) -RelayZones(5); 0 -RelayZones(5)]"  fs=32*60
  ZC   1 : elements/ZC     typez=Free expression  z1="[0  0; RelayZones(1) 0; RelayZones(1) RelayZones(1); 0 RelayZones(1)]"  z2="[0  0; RelayZones(2) 0; RelayZones(2) RelayZones(2); 0 RelayZones(2)]"  z3="[0  0; RelayZones(3) 0; RelayZones(3) RelayZones(3); 0 RelayZones(3)]"  z4="[0  0; RelayZones(4) 0; RelayZones(4) RelayZones(4); 0 RelayZones(4)]"  zr="[0  0; -RelayZones(5) 0; -RelayZones(5) -RelayZones(5); 0 -RelayZones(5)]"  fs=32*60
  I : Outport
  II : Outport  Port=2
  III : Outport  Port=3
  IV : Outport  Port=4
  CS : Outport  Port=5
  tag scope: ZC=global, faultC=global
  wires:
  BM/1 -> " "/1
  BM/2 -> " 1"/1
  BM/3 -> " 5"/1
  V:phasor/1 -> BM/1
  I: phasor/1 -> BM/2
  BM/4 -> ZC   1/1, [ZC], "ZC   "/1
  ZC   1/2 -> " 2"/1
  ZC   1/3 -> " 3"/1
  ZC   1/4 -> " 4"/1
  ZC   1/5 -> " 6"/1
  "2 "/1 -> II/1, 3/1
  3/1 -> 4/1, III/1
  4/1 -> IV/1
  "ZC   "/5 -> CS/1
  "ZC   "/4 -> 4/2
  "ZC   "/3 -> 3/2
  "ZC   "/2 -> "2 "/2
  "ZC   "/1 -> "2 "/1, I/1
  ZC   1/1 -> [faultC]

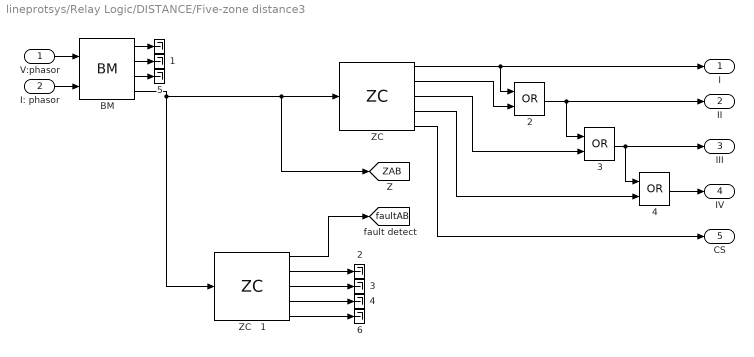
== system lineprotsys/Relay Logic/DISTANCE/Five-zone distance3 ==
  V:phasor : Inport
  I: phasor : Inport  Port=2
   {,1..6} (7 alike) : Terminator
  "2 " : Logic  Operator=OR
  3 : Logic  Operator=OR
  4 : Logic  Operator=OR
  BM : elements/BM  tpostv=none  plenv=4  tposti=none  pleni=4  tposts=none  plens=4  tpostz=none  plenz=4
  "ZC   " : elements/ZC     typez=Free expression  z1="[0  0; RelayZones(1) 0; RelayZones(1) RelayZones(1); 0 RelayZones(1)]"  z2="[0  0; RelayZones(2) 0; RelayZones(2) RelayZones(2); 0 RelayZones(2)]"  z3="[0  0; RelayZones(3) 0; RelayZones(3) RelayZones(3); 0 RelayZones(3)]"  z4="[0  0; RelayZones(4) 0; RelayZones(4) RelayZones(4); 0 RelayZones(4)]"  zr="[0  0; -RelayZones(5) 0; -RelayZones(5) -RelayZones(5); 0 -RelayZones(5)]"  fs=32*60
  ZC   1 : elements/ZC     typez=Free expression  z1="[0  0; RelayZones(1) 0; RelayZones(1) RelayZones(1); 0 RelayZones(1)]"  z2="[0  0; RelayZones(2) 0; RelayZones(2) RelayZones(2); 0 RelayZones(2)]"  z3="[0  0; RelayZones(3) 0; RelayZones(3) RelayZones(3); 0 RelayZones(3)]"  z4="[0  0; RelayZones(4) 0; RelayZones(4) RelayZones(4); 0 RelayZones(4)]"  zr="[0  0; -RelayZones(5) 0; -RelayZones(5) -RelayZones(5); 0 -RelayZones(5)]"  fs=32*60
  I : Outport
  II : Outport  Port=2
  III : Outport  Port=3
  IV : Outport  Port=4
  CS : Outport  Port=5
  tag scope: ZAB=global, faultAB=global
  wires:
  BM/1 -> " "/1
  BM/2 -> " 1"/1
  BM/3 -> " 5"/1
  V:phasor/1 -> BM/1
  I: phasor/1 -> BM/2
  BM/4 -> ZC   1/1, [ZAB], "ZC   "/1
  ZC   1/2 -> " 2"/1
  ZC   1/3 -> " 3"/1
  ZC   1/4 -> " 4"/1
  ZC   1/5 -> " 6"/1
  "2 "/1 -> II/1, 3/1
  3/1 -> 4/1, III/1
  4/1 -> IV/1
  "ZC   "/5 -> CS/1
  "ZC   "/4 -> 4/2
  "ZC   "/3 -> 3/2
  "ZC   "/2 -> "2 "/2
  "ZC   "/1 -> "2 "/1, I/1
  ZC   1/1 -> [faultAB]

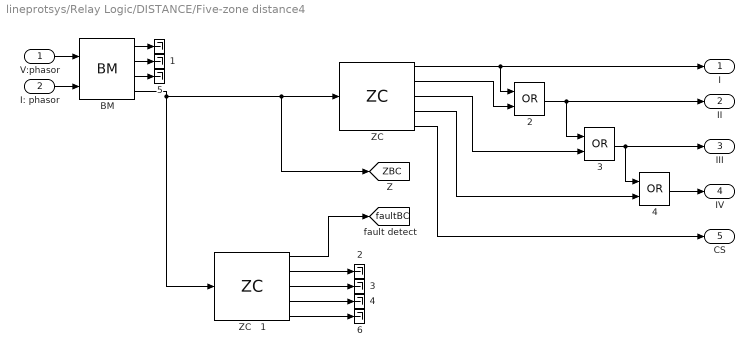
== system lineprotsys/Relay Logic/DISTANCE/Five-zone distance4 ==
  V:phasor : Inport
  I: phasor : Inport  Port=2
   {,1..6} (7 alike) : Terminator
  "2 " : Logic  Operator=OR
  3 : Logic  Operator=OR
  4 : Logic  Operator=OR
  BM : elements/BM  tpostv=none  plenv=4  tposti=none  pleni=4  tposts=none  plens=4  tpostz=none  plenz=4
  "ZC   " : elements/ZC     typez=Free expression  z1="[0  0; RelayZones(1) 0; RelayZones(1) RelayZones(1); 0 RelayZones(1)]"  z2="[0  0; RelayZones(2) 0; RelayZones(2) RelayZones(2); 0 RelayZones(2)]"  z3="[0  0; RelayZones(3) 0; RelayZones(3) RelayZones(3); 0 RelayZones(3)]"  z4="[0  0; RelayZones(4) 0; RelayZones(4) RelayZones(4); 0 RelayZones(4)]"  zr="[0  0; -RelayZones(5) 0; -RelayZones(5) -RelayZones(5); 0 -RelayZones(5)]"  fs=32*60
  ZC   1 : elements/ZC     typez=Free expression  z1="[0  0; RelayZones(1) 0; RelayZones(1) RelayZones(1); 0 RelayZones(1)]"  z2="[0  0; RelayZones(2) 0; RelayZones(2) RelayZones(2); 0 RelayZones(2)]"  z3="[0  0; RelayZones(3) 0; RelayZones(3) RelayZones(3); 0 RelayZones(3)]"  z4="[0  0; RelayZones(4) 0; RelayZones(4) RelayZones(4); 0 RelayZones(4)]"  zr="[0  0; -RelayZones(5) 0; -RelayZones(5) -RelayZones(5); 0 -RelayZones(5)]"  fs=32*60
  I : Outport
  II : Outport  Port=2
  III : Outport  Port=3
  IV : Outport  Port=4
  CS : Outport  Port=5
  tag scope: ZBC=global, faultBC=global
  wires:
  BM/1 -> " "/1
  BM/2 -> " 1"/1
  BM/3 -> " 5"/1
  V:phasor/1 -> BM/1
  I: phasor/1 -> BM/2
  BM/4 -> ZC   1/1, [ZBC], "ZC   "/1
  ZC   1/2 -> " 2"/1
  ZC   1/3 -> " 3"/1
  ZC   1/4 -> " 4"/1
  ZC   1/5 -> " 6"/1
  "2 "/1 -> II/1, 3/1
  3/1 -> 4/1, III/1
  4/1 -> IV/1
  "ZC   "/5 -> CS/1
  "ZC   "/4 -> 4/2
  "ZC   "/3 -> 3/2
  "ZC   "/2 -> "2 "/2
  "ZC   "/1 -> "2 "/1, I/1
  ZC   1/1 -> [faultBC]

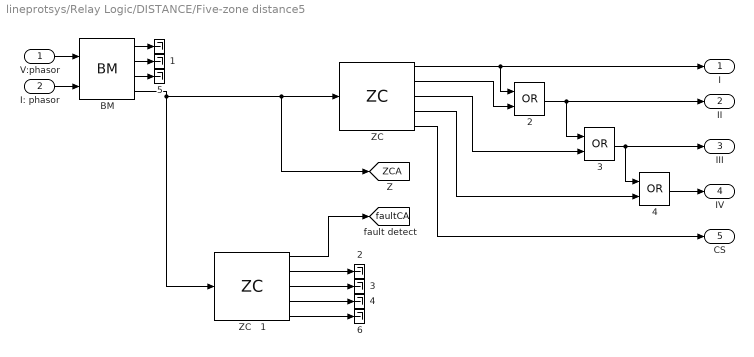
== system lineprotsys/Relay Logic/DISTANCE/Five-zone distance5 ==
  V:phasor : Inport
  I: phasor : Inport  Port=2
   {,1..6} (7 alike) : Terminator
  "2 " : Logic  Operator=OR
  3 : Logic  Operator=OR
  4 : Logic  Operator=OR
  BM : elements/BM  tpostv=none  plenv=4  tposti=none  pleni=4  tposts=none  plens=4  tpostz=none  plenz=4
  "ZC   " : elements/ZC     typez=Free expression  z1="[0  0; RelayZones(1) 0; RelayZones(1) RelayZones(1); 0 RelayZones(1)]"  z2="[0  0; RelayZones(2) 0; RelayZones(2) RelayZones(2); 0 RelayZones(2)]"  z3="[0  0; RelayZones(3) 0; RelayZones(3) RelayZones(3); 0 RelayZones(3)]"  z4="[0  0; RelayZones(4) 0; RelayZones(4) RelayZones(4); 0 RelayZones(4)]"  zr="[0  0; -RelayZones(5) 0; -RelayZones(5) -RelayZones(5); 0 -RelayZones(5)]"  fs=32*60
  ZC   1 : elements/ZC     typez=Free expression  z1="[0  0; RelayZones(1) 0; RelayZones(1) RelayZones(1); 0 RelayZones(1)]"  z2="[0  0; RelayZones(2) 0; RelayZones(2) RelayZones(2); 0 RelayZones(2)]"  z3="[0  0; RelayZones(3) 0; RelayZones(3) RelayZones(3); 0 RelayZones(3)]"  z4="[0  0; RelayZones(4) 0; RelayZones(4) RelayZones(4); 0 RelayZones(4)]"  zr="[0  0; -RelayZones(5) 0; -RelayZones(5) -RelayZones(5); 0 -RelayZones(5)]"  fs=32*60
  I : Outport
  II : Outport  Port=2
  III : Outport  Port=3
  IV : Outport  Port=4
  CS : Outport  Port=5
  tag scope: ZCA=global, faultCA=global
  wires:
  BM/1 -> " "/1
  BM/2 -> " 1"/1
  BM/3 -> " 5"/1
  V:phasor/1 -> BM/1
  I: phasor/1 -> BM/2
  BM/4 -> ZC   1/1, [ZCA], "ZC   "/1
  ZC   1/2 -> " 2"/1
  ZC   1/3 -> " 3"/1
  ZC   1/4 -> " 4"/1
  ZC   1/5 -> " 6"/1
  "2 "/1 -> II/1, 3/1
  3/1 -> 4/1, III/1
  4/1 -> IV/1
  "ZC   "/5 -> CS/1
  "ZC   "/4 -> 4/2
  "ZC   "/3 -> 3/2
  "ZC   "/2 -> "2 "/2
  "ZC   "/1 -> "2 "/1, I/1
  ZC   1/1 -> [faultCA]

== system lineprotsys/Relay Logic/Power Swing/Subsystem ==
  Z1 : Inport
  Z2 : Inport  Port=2
  2 : RelationalOperator  OutDataTypeStr=boolean  RndMeth=Nearest
  Clock: Tz1 : Clock
  Clock: Tz2 : Clock
  Data Store Memory : DataStoreMemory  DataStoreName=TZ1  ReadBeforeWriteMsg=warning  WriteAfterWriteMsg=warning  WriteAfterReadMsg=warning  ShowAdditionalParam=off
  Data Store Memory1 : DataStoreMemory  DataStoreName=TZ2  ReadBeforeWriteMsg=warning  WriteAfterWriteMsg=warning  WriteAfterReadMsg=warning  ShowAdditionalParam=off
  Data Store Write : DataStoreWrite  DataStoreName=TZ1
  Data Store Write1 : DataStoreWrite  DataStoreName=TZ2
  Initial : Constant  Value=0
  Initial1 : Constant  Value=Tswing
  Sum : Sum  Inputs=|+-
  Switch : Switch
  Switch1 : Switch
  Switch2 : Switch
  Tz1 : DataStoreRead  DataStoreName=TZ1
  Tz2 : DataStoreRead  DataStoreName=TZ1
  block : Outport
  wires:
  Clock: Tz1/1 -> Switch/3
  Switch/1 -> Switch/1, Data Store Write/1
  Clock: Tz2/1 -> Switch1/3
  Switch1/1 -> Switch1/1, Data Store Write1/1
  Z2/1 -> Switch1/2
  Tz1/1 -> Sum/1
  Tz2/1 -> Sum/2
  Sum/1 -> Switch2/1
  Initial/1 -> Switch2/3
  Z1/1 -> Switch2/2, Switch/2
  2/1 -> block/1
  Switch2/1 -> 2/1
  Initial1/1 -> 2/2

== system lineprotsys/Relay Logic/Power Swing/Z: power swing ==
  Z : Inport
  Demux : Demux  Outputs=5
  S-Function : S-Function  FunctionName=zc2  Parameters=z1,z2,z3,z4,zr,typez,fs,n,minx,flagc,m,b  SFunctionDeploymentMode=off  EnableBusSupport=off
  1 : Outport  InitialOutput=0
  2 : Outport  Port=2  InitialOutput=0
  3 : Outport  Port=3  InitialOutput=0
  4 : Outport  Port=4  InitialOutput=0
  R : Outport  Port=5  InitialOutput=0
  wires:
  Demux/5 -> R/1
  Z/1 -> S-Function/1
  Demux/4 -> 4/1
  Demux/3 -> 3/1
  Demux/2 -> 2/1
  Demux/1 -> 1/1
  S-Function/1 -> Demux/1
